simulink model "slapp"  (R2024b)
settings: Solver=FixedStepAuto  StartTime=0.0  StopTime=20  RelTol=1e-3
libraries: spikertlib x18
settings Model: Creator=ymatsuur  LastModifiedBy=yokano
settings OptimizationCC: DefaultParameterBehavior=Inlined  EnhancedBackFolding=on  PassReuseOutputArgsAs=Individual arguments  ZeroExternalMemoryAtStartup=off  ZeroInternalMemoryAtStartup=off  OptimizeBlockOrder=speed  DifferentSizesBufferReuse=on  OptimizationCustomize=off  EfficientTunableParamExpr=on
settings DebuggingCC: ParameterTunabilityLossMsg=error
settings HardwareCC: ProdBitPerPointer=32  ProdBitPerSizeT=32  ProdBitPerPtrDiffT=32  ProdLargestAtomicInteger=Long  ProdLargestAtomicFloat=Double  ProdWordSize=32  ProdHWDeviceType=ARM Compatible->ARM Cortex-M
settings SFSimCC: MATLABDynamicMemAlloc=off
settings RTWCC: Description=Embedded Coder  SystemTargetFile=ert.tlc  GenCodeOnly=on  TemplateMakefile=ert_default_tmf  GPUComputeCapability=3.5
settings CodeAppCC: ForceParamTrailComments=on  IgnoreCustomStorageClasses=off  OperatorAnnotations=on  SimulinkDataObjDesc=on  SFDataObjDesc=on  InsertBlockDesc=on
settings ERTTargetCC: TargetLangStandard=C99 (ISO)  GenerateSampleERTMain=on  IncludeMdlTerminateFcn=off  ERTCustomFileTemplate=addspikertmain.tlc  ERTFilePackagingFormat=Compact  DynamicArrayContainerType=coder::array
settings ConfigComp: DVMode=DesignErrorDetection  DVTestSuiteOptimization=Auto  DVDefectChecker=off  DVDetectOutOfBounds=on  DVModelReferenceHarness=on  DVHarnessSource=Signal Editor

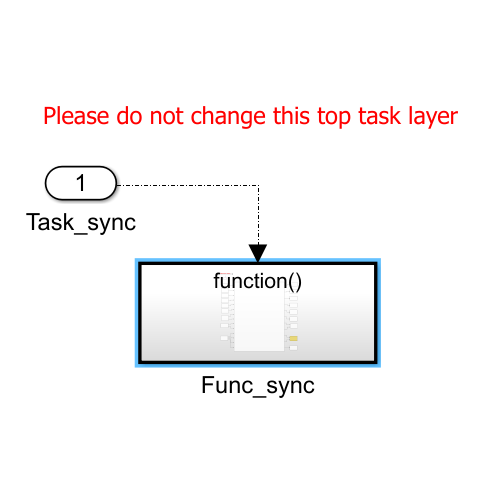
[thumbnail: Simulink's stored preview of the top-level diagram]
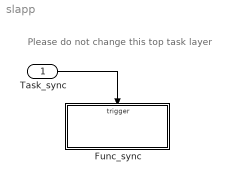
== system slapp ==
  note: Please do not change this top task layer
  Task_sync : Inport  OutputFunctionCall=on
  Func_sync : Subsystem  TreatAsAtomicUnit=on
  wires:
  Task_sync/1 -> Func_sync/Trigger

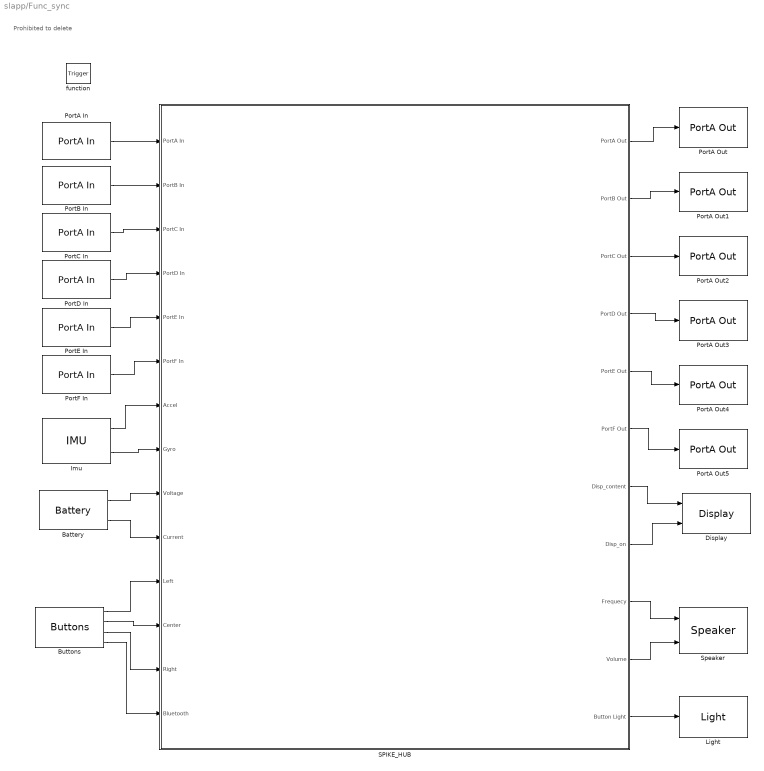
== system slapp/Func_sync ==
  note: Prohibited to delete
  function : TriggerPort  TriggerType=function-call  VariantControl=(inherit)
  Battery : spikertlib/Large hub/Battery
  Buttons : spikertlib/Large hub/Buttons
  Display : spikertlib/Large hub/Display  Mode=Numeric  UpOrientation=RIGHT
  Imu : spikertlib/Large hub/IMU
  Light : spikertlib/Large hub/Light
  PortA In : spikertlib/Powered Up device/PortA In  PortID=A  SensorType=Force  SensorMode=Reflection  LightOn=on
  PortA Out : spikertlib/Powered Up device/PortA Out  PortID=A  Mode=None  EncorderReset=No reset  Direction=Clockwise
      settings: AttributesFormatString=|
      | PortID = %<PortID>
      | Mode = %<Mode>
  PortA Out1 : spikertlib/Powered Up device/PortA Out  PortID=B  Mode=Set the power [%]  EncorderReset=Reset  Direction=Clockwise
      settings: AttributesFormatString=|
      | PortID = %<PortID>
      | Mode = %<Mode>
  PortA Out2 : spikertlib/Powered Up device/PortA Out  PortID=C  Mode=Set the power [%]  EncorderReset=Reset  Direction=Couter-clockwise
      settings: AttributesFormatString=|
      | PortID = %<PortID>
      | Mode = %<Mode>
  PortA Out3 : spikertlib/Powered Up device/PortA Out  PortID=D  Mode=None  EncorderReset=No reset  Direction=Clockwise
      settings: AttributesFormatString=|
      | PortID = %<PortID>
      | Mode = %<Mode>
  PortA Out4 : spikertlib/Powered Up device/PortA Out  PortID=E  Mode=None  EncorderReset=No reset  Direction=Clockwise
      settings: AttributesFormatString=|
      | PortID = %<PortID>
      | Mode = %<Mode>
  PortA Out5 : spikertlib/Powered Up device/PortA Out  PortID=F  Mode=None  EncorderReset=No reset  Direction=Clockwise
      settings: AttributesFormatString=|
      | PortID = %<PortID>
      | Mode = %<Mode>
  PortB In : spikertlib/Powered Up device/PortA In  PortID=B  SensorType=Motor  SensorMode=Reflection  LightOn=on
  PortC In : spikertlib/Powered Up device/PortA In  PortID=C  SensorType=Motor  SensorMode=Reflection  LightOn=on
  PortD In : spikertlib/Powered Up device/PortA In  PortID=D  SensorType=Ultrasonic  SensorMode=Reflection  LightOn=on
  PortE In : spikertlib/Powered Up device/PortA In  PortID=E  SensorType=Color  SensorMode=Reflection  LightOn=on
  PortF In : spikertlib/Powered Up device/PortA In  PortID=F  SensorType=None  SensorMode=Reflection  LightOn=on
  SPIKE_HUB : Subsystem  TreatAsAtomicUnit=on
      mask Display: image(['sphub.png']);
  Speaker : spikertlib/Large hub/Speaker
  wires:
  Imu/1 -> SPIKE_HUB/7(Accel)
  Imu/2 -> SPIKE_HUB/8(Gyro)
  Battery/1 -> SPIKE_HUB/9(Voltage)
  PortA In/1 -> SPIKE_HUB/1(PortA In)
  PortB In/1 -> SPIKE_HUB/2(PortB In)
  PortD In/1 -> SPIKE_HUB/4(PortD In)
  PortC In/1 -> SPIKE_HUB/3(PortC In)
  PortE In/1 -> SPIKE_HUB/5(PortE In)
  PortF In/1 -> SPIKE_HUB/6(PortF In)
  Buttons/1 -> SPIKE_HUB/11(Left)
  Buttons/2 -> SPIKE_HUB/12(Center)
  Buttons/3 -> SPIKE_HUB/13(Right)
  Buttons/4 -> SPIKE_HUB/14(Bluetooth)
  SPIKE_HUB/1(PortA Out) -> PortA Out/1
  SPIKE_HUB/2(PortB Out) -> PortA Out1/1
  SPIKE_HUB/3(PortC Out) -> PortA Out2/1
  SPIKE_HUB/4(PortD Out) -> PortA Out3/1
  SPIKE_HUB/5(PortE Out) -> PortA Out4/1
  SPIKE_HUB/6(PortF Out) -> PortA Out5/1
  SPIKE_HUB/7(Disp_content) -> Display/1
  SPIKE_HUB/11(Button Light) -> Light/1
  SPIKE_HUB/9(Frequecy) -> Speaker/1
  Battery/2 -> SPIKE_HUB/10(Current)
  SPIKE_HUB/10(Volume) -> Speaker/2
  SPIKE_HUB/8(Disp_on) -> Display/2

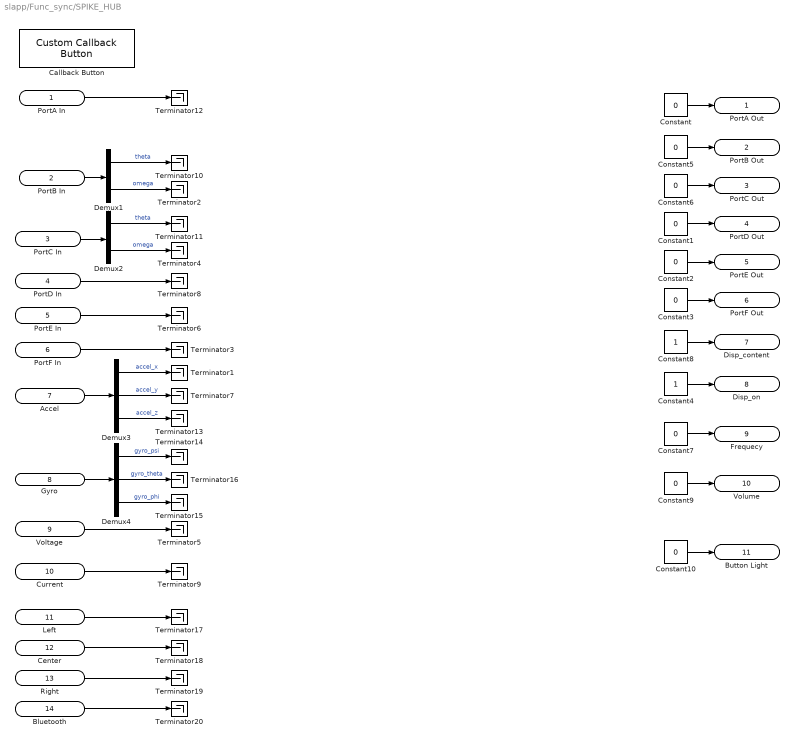
== system slapp/Func_sync/SPIKE_HUB ==
  PortA In : Inport
  PortB In : Inport  Port=2
  PortC In : Inport  Port=3
  PortD In : Inport  Port=4
  PortE In : Inport  Port=5
  PortF In : Inport  Port=6
  Accel : Inport  Port=7
  Gyro : Inport  Port=8
  Voltage : Inport  Port=9
  Current : Inport  Port=10
  Left : Inport  Port=11
  Center : Inport  Port=12
  Right : Inport  Port=13
  Bluetooth : Inport  Port=14
  Callback Button : CustomCallbackButton  Description=Generate and build code. write executable to SPIKE  Configuration="{\"components\":[{\"name\":\"BackgroundImageComponent\",\"settings\":{\"image\":{\"size\":[0,0],\"src\":\"default\",\"srcOrientation\":\"Right\"},\"position\":[0,0,1,1]}},{\"name\":\"ButtonStateComponent\",\"settings\":{\"buttonType\":\"momentary\",\"clickFcn\":\"controlsetupspikert_callback;\\ncopyspikert(2)\\ncopyspikert(3)\",\"latched\":false,\"offValue\":null,\"onValue\":1,\"position\":[0,0,1,1],\"pressDelay\":\"500\",\"pressFcn\":\"\",\"repeatInterval\":\"0\",\"states\":[{\"horizontalAlignment\":\"center\",\"image\":{\"position\":[0,0,1,1],\"size\":[1,1],\"src\":\"default\",\"srcOrientation\":\"Right\"},\"label\":{\"color\":[1,1,1],\"icon\":{\"size\":[0,0],\"src\":\"default\",\"srcOrientation\":\"Right\"},\"iconOffset\":0,\"iconPlacement\":\"left\",\"opacity\":1,\"show\":true,\"text\":{\"content\":\"Build & Write\",\"font\":\"Helvetica\"}},\"labelOffset\":[0,0],\"verticalAlignment\":\"middle\"},{\"horizontalAlignment\":\"center\",\"image\":{\"position\":[0,0,1,1],\"size\":[1,1],\"src\":\"default\",\"srcOrientation\":\"Right\"},\"label\":{\"color\":[0.01176470588,0.01176470588,0.01176470588,1],\"icon\":{\"size\":[0,0],\"src\":\"default\",\"srcOrientation\":\"Right\"},\"iconOffset\":0,\"iconPlacement\":\"left\",\"opacity\":1,\"show\":true,\"text\":{\"content\":\"Build & Write\",\"font\":\"Helvetica\"}},\"labelOffset\":[0,0],\"verticalAlignment\":\"middle\"},{\"horizontalAlignment\":\"center\",\"image\":{\"position\":[0,0,1,1],\"size\":[1,1],\"src\":\"default\",\"srcOrientation\":\"Right\"},\"label\":{\"color\":[0.01176470588,0.01176470588,0.01176470588,1],\"icon\":{\"size\":[0,0],\"src\":\"default\",\"srcOrientation\":\"Right\"},\"iconOffset\":0,\"iconPlacement\":\"left\",\"opacity\":1,\"show\":true,\"text\":{\"content\":\"Build & Write\",\"font\":\"Helvetica\"}},\"labelOffset\":[0,0],\"verticalAlignment\":\"middle\"},{\"horizontalAlignment\":\"center\",\"image\":{\"position\":[0,0,1,1],\"size\":[1,1],\"src\":\"default\",\"srcOrientation\":\"Right\"},\"label\":{\"color\":[0.01176470588,0.01176470588,0.01176470588,1],\"icon\":{\"size\":[0,0],\"src\":\"default\",\"srcOrientation\":\"Right\"},\"iconOffset\":0,\"iconPlacement\":\"left\",\"opacity\":1,\"show\":true,\"text\":{\"content\":\"Build & Write\",\"font\":\"Helvetica\"}},\"labelOffset\":[0,0],\"verticalAlignment\":\"middle\"}]}},{\"name\":\"ForegroundImageComponent\",\"settings\":{\"image\":{\"size\":[0,0],\"src\":\"default\",\"srcOrientation\":\"Right\"},\"isForeground\":1,\"position\":[0,0,1,1]}}],\"settings\":{\"BindingType\":\"standalone\",\"backgroundColor\":[244,244,244,1],\"backgroundOffset\":0.2,\"backgroundOpacity\":1,\"fixedAspectRatio\":\"off\",\"foregroundColor\":[0.01176470588,0.01176470588,0.01176470588,1],\"migratedFromLegacy\":true,\"useBackgroundColor\":true,\"variant\":\"callback\",\"version\":\"R2023a\"},\"type\":\"Button\"}"  CustomBackgroundColor="{\"color\":[0.8509803921568627,0.3254901960784314,0.09803921568627451],\"show\":true}"
  Constant{,1..3,5..7,9..10} (9 alike) : Constant  Value=0
  Constant4 : Constant
  Constant8 : Constant
  Demux1 : Demux  Outputs=2
  Demux2 : Demux  Outputs=2
  Demux3 : Demux  Outputs=3
  Demux4 : Demux  Outputs=3
  Terminator{1..20} (20 alike) : Terminator
  PortA Out : Outport
  PortB Out : Outport  Port=2
  PortC Out : Outport  Port=3
  PortD Out : Outport  Port=4
  PortE Out : Outport  Port=5
  PortF Out : Outport  Port=6
  Disp_content : Outport  Port=7
  Disp_on : Outport  Port=8
  Frequecy : Outport  Port=9
  Volume : Outport  Port=10
  Button Light : Outport  Port=11
  wires:
  Demux3/1 -> Terminator1/1  "accel_x"
  PortF In/1 -> Terminator3/1
  Demux1/2 -> Terminator2/1  "omega"
  Demux1/1 -> Terminator10/1  "theta"
  PortB In/1 -> Demux1/1
  Demux2/1 -> Terminator11/1  "theta"
  Demux2/2 -> Terminator4/1  "omega"
  PortC In/1 -> Demux2/1
  Accel/1 -> Demux3/1
  Demux3/2 -> Terminator7/1  "accel_y"
  Demux3/3 -> Terminator13/1  "accel_z"
  Demux4/3 -> Terminator15/1  "gyro_phi"
  Demux4/2 -> Terminator16/1  "gyro_theta"
  Gyro/1 -> Demux4/1
  Demux4/1 -> Terminator14/1  "gyro_psi"
  Left/1 -> Terminator17/1
  Center/1 -> Terminator18/1
  Right/1 -> Terminator19/1
  Bluetooth/1 -> Terminator20/1
  Constant/1 -> PortA Out/1
  Constant2/1 -> PortE Out/1
  Constant3/1 -> PortF Out/1
  Constant4/1 -> Disp_on/1
  Constant10/1 -> Button Light/1
  Constant1/1 -> PortD Out/1
  Constant7/1 -> Frequecy/1
  Voltage/1 -> Terminator5/1
  PortE In/1 -> Terminator6/1
  PortD In/1 -> Terminator8/1
  Constant8/1 -> Disp_content/1
  Current/1 -> Terminator9/1
  Constant9/1 -> Volume/1
  PortA In/1 -> Terminator12/1
  Constant5/1 -> PortB Out/1
  Constant6/1 -> PortC Out/1
